simulink subsystem "Direct_Thrust_Command"  (R2023a)
settings: Solver=VariableStepAuto  StartTime=0.0  StopTime=10.0  RelTol=1e-3
settings Model: Creator=thesa  LastModifiedBy=thesa

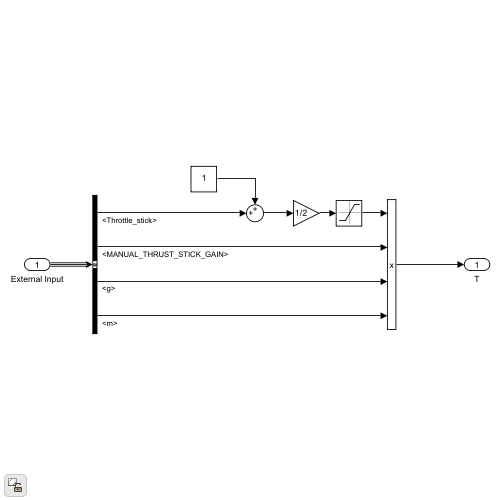
[thumbnail: Simulink's stored preview of the top-level diagram]
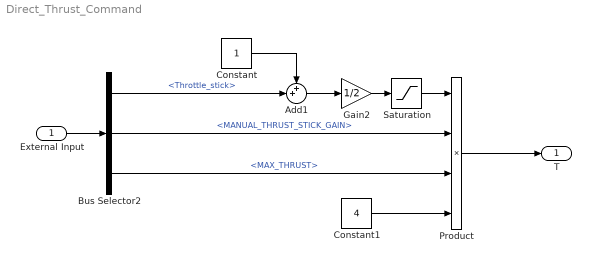
== system Direct_Thrust_Command ==
  External Input : Inport
  Add1 : Sum  Inputs=++|
  Bus Selector2 : BusSelector  OutputSignals=Pilot Input.Sticks.Throttle_stick,Pilot Input.Parameters.MANUAL_THRUST_STICK_GAIN,Vehicle Parameters.MAX_THRUST
  Constant : Constant
  Constant1 : Constant  Value=4
  Gain2 : Gain  Gain=1/2
  Product : Product  Inputs=4
  Saturation : Saturate  UpperLimit=1  LowerLimit=0
  T : Outport
  wires:
  External Input/1 -> Bus Selector2/1
  Bus Selector2/1 -> Add1/2  "<Throttle_stick>"
  Add1/1 -> Gain2/1
  Constant/1 -> Add1/1
  Bus Selector2/2 -> Product/2  "<MANUAL_THRUST_STICK_GAIN>"
  Gain2/1 -> Saturation/1
  Bus Selector2/3 -> Product/3  "<MAX_THRUST>"
  Saturation/1 -> Product/1
  Constant1/1 -> Product/4
  Product/1 -> T/1
